simulink model "GFM_parallel_alt"  (R2024a)
settings: Solver=VariableStepAuto  StartTime=0.0  StopTime=40  FixedStep=5e-6  RelTol=1e-3
values from neighbouring files (symbols this model uses):
  Cf_pu = 0.03    [main__gfm.m]    (also in main_parallel.m; main_parallel_alt.m; main_standalone.m; scr.m)
  Cs_pu = 0.3    [main_parallel.m]    (also in main_parallel_alt.m; main_standalone.m)
  Dp = 0.02    [main__gfm.m]    (also in main_parallel.m; main_parallel_alt.m; main_standalone.m; scr.m)
  Dp1 = Dp    (= 0.02)    [main_parallel.m]    (also in main_parallel_alt.m)
  Dp2 = Dp    (= 0.02)    [main_parallel.m]    (also in main_parallel_alt.m)
  Dq = 0.3    [main__gfm.m]    (also in main_parallel.m; main_parallel_alt.m; main_standalone.m; scr.m)
  Dq1 = Dq    (= 0.3)    [main_parallel.m]    (also in main_parallel_alt.m)
  Dq2 = Dq    (= 0.3)    [main_parallel.m]    (also in main_parallel_alt.m)
  fac = 0    [main__gfm.m]    (also in main_parallel.m; main_parallel_alt.m; main_standalone.m; scr.m)
  H = 1.2    [main__gfm.m]    (also in main_parallel.m = 0.3; main_parallel_alt.m = 0.3; main_standalone.m; scr.m)
  I_load = Vpcc0/Zload_pu    [main__gfm.m]    (also in main_parallel.m = Vpcc/Zload_pu; main_parallel_alt.m = Vpoc/Zload_pu; main_standalone.m; scr.m)
  Ic1 = (Vconv1-Vlcl1)/(Rc_pu+1i*Lc_pu)    [main_parallel.m]    (also in main_parallel_alt.m = (Vconv1-Vpcc1)/(Rc_pu+1i*Lc_pu))
  Ic2 = (Vconv2-Vlcl2)/(Rc_pu+1i*Lc_pu)    [main_parallel.m]    (also in main_parallel_alt.m = (Vconv2-Vpcc2)/(Rc_pu+1i*Lc_pu))
  If1 = (Vlcl1-Vpcc)/(Rgf_pu+1i*Lgf_pu)    [main_parallel.m]    (also in main_parallel_alt.m = (Vpcc1-Vpoc)/(Rgf_pu+1i*Lgf_pu))
  If2 = (Vlcl2-Vpcc)/(Rgf_pu+1i*Lgf_pu)    [main_parallel.m]    (also in main_parallel_alt.m = (Vpcc2-Vpoc)/(Rgf_pu+1i*Lgf_pu))
  Iinf = (Vpcc-Vinf)/(Rgrid_pu+1i*Lgrid_pu)    [main_parallel.m]    (also in main_parallel_alt.m = (Vpoc-Vinf)/(Rgrid_pu+1i*Lgrid_pu))
  Kd = 50    [main__gfm.m]    (also in main_parallel.m; main_parallel_alt.m = 100; main_standalone.m; scr.m)
  kfi = 0    [main__gfm.m]    (also in main_parallel.m; main_parallel_alt.m; main_standalone.m; scr.m)
  kii = Rc_pu / L * kpi    [main__gfm.m]    (also in main_parallel.m; main_parallel_alt.m; main_standalone.m; scr.m)
  kiq = 0.1    [main__gfm.m]    (also in main_parallel.m = 0.01; main_parallel_alt.m = 0.01; main_standalone.m; scr.m)
  kivd = 100    [main__gfm.m]    (also in main_parallel.m = 50; main_parallel_alt.m = 50; main_standalone.m; scr.m)
  kivq = 100    [main__gfm.m]    (also in main_parallel.m = 50; main_parallel_alt.m = 50; main_standalone.m; scr.m)
  kpi = 2 * pi * f_bw * L    [main__gfm.m]    (also in main_parallel.m; main_parallel_alt.m; main_standalone.m; scr.m)
  kpvd = 0.1    [main__gfm.m]    (also in main_parallel.m = 0.45; main_parallel_alt.m = 0.45; main_standalone.m; scr.m)
  kpvq = 0.1    [main__gfm.m]    (also in main_parallel.m = 0.45; main_parallel_alt.m = 0.45; main_standalone.m; scr.m = 1)
  Lc_pu = Lc / Lb    [main__gfm.m]    (also in main_parallel.m; main_parallel_alt.m; main_standalone.m; scr.m)
  Lgf_pu = Lgf/Lb    (= 0.0166666666667)    [main_parallel.m]    (also in main_parallel_alt.m; main_standalone.m)
  Lgrid_pu = 1    [main_parallel.m]    (also in main_parallel_alt.m)
  Pref1 = -line_flow(7,4)    [main_parallel.m]    (also in main_parallel_alt.m)
  Pref2 = -line_flow(3,4)    [main_parallel.m]    (also in main_parallel_alt.m)
  PsiId1 = real(Vconv_c1)-real(Vpcc_c)+X*imag(Ifc1)    [main_parallel.m]    (also in main_parallel_alt.m)
  PsiId2 = real(Vconv_c2)-real(Vpcc_c)+X*imag(Ifc2)    [main_parallel.m]    (also in main_parallel_alt.m)
  PsiIq1 = imag(Vconv_c1)-imag(Vpcc_c)-X*real(Ifc1)    [main_parallel.m]    (also in main_parallel_alt.m)
  PsiIq2 = imag(Vconv_c2)-imag(Vpcc_c)-X*real(Ifc2)    [main_parallel.m]    (also in main_parallel_alt.m)
  PsiP1 = real(Ifc1)-wCpu*imag(Vpcc_c)*fac+imag(Ifc1)*kfi    [main_parallel.m]    (also in main_parallel_alt.m)
  PsiP2 = real(Ifc2)-wCpu*imag(Vpcc_c)*fac+imag(Ifc2)*kfi    [main_parallel.m]    (also in main_parallel_alt.m)
  PsiV1 = imag(Ifc1)+wCpu*real(Vpcc_c)*fac+real(Ifc1)*kfi    [main_parallel.m]    (also in main_parallel_alt.m)
  PsiV2 = imag(Ifc2)+wCpu*real(Vpcc_c)*fac+real(Ifc2)*kfi    [main_parallel.m]    (also in main_parallel_alt.m)
  Qref1 = -line_flow(7,5)    [main_parallel.m]    (also in main_parallel_alt.m)
  Qref2 = -line_flow(3,5)    [main_parallel.m]    (also in main_parallel_alt.m)
  Rc_pu = Rc / Zb    (= 5.19390581717e-06)    [main__gfm.m]    (also in main_parallel.m; main_parallel_alt.m; main_standalone.m; scr.m)
  Rf_pu = Rf / Zb    [main__gfm.m]    (also in main_parallel.m; main_parallel_alt.m; main_standalone.m; scr.m)
  Rgf_pu = 0    [main_parallel.m]    (also in main_parallel_alt.m)
  Rgrid_pu = Lgrid_pu*XrXg    (= 0)    [main_parallel.m]    (also in main_parallel_alt.m)
  Rs_pu = 0.1    [main_parallel.m]    (also in main_parallel_alt.m; main_standalone.m)
  theta_ref = theta(2,1)    [main__gfm.m]    (also in main_parallel.m = theta(3,1); main_parallel_alt.m = theta(3,1); main_standalone.m = theta(3,1); scr.m)
  Vcf1 = Vlcl1+ Rf_pu*Icf1    [main_parallel.m]    (also in main_parallel_alt.m = Vpcc1+ Rf_pu*Icf1)
  Vcf2 = Vlcl2+ Rf_pu*Icf2    [main_parallel.m]    (also in main_parallel_alt.m = Vpcc2+ Rf_pu*Icf2)
  Vconv1 = V0(1,1)    [main_parallel.m]    (also in main_parallel_alt.m)
  Vconv_c1 = Vconv1 * exp(-1i*theta_ref)    [main_parallel.m]    (also in main_parallel_alt.m)
  Vconv_c2 = Vconv2 * exp(-1i*theta_ref)    [main_parallel.m]    (also in main_parallel_alt.m)
  Vinf = V0(3,1)    [main__gfm.m]    (also in main_parallel.m = V0(6,1); main_parallel_alt.m = V0(6,1); main_standalone.m = V0(4,1); scr.m)
  Vpcc = V0(3,1)    [main_parallel.m]
  Vs = Vpcc + Rs_pu*Igf    [main_parallel.m]    (also in main_parallel_alt.m = Vpoc + Rs_pu*Igf; main_standalone.m = Vload+Rs_pu*Ibf)
  wCpu = Zb * wb * Cf    (= 0.03)    [main__gfm.m]    (also in main_parallel.m; main_parallel_alt.m; main_standalone.m; scr.m)
  wLpu = X    [main__gfm.m]    (also in main_parallel.m; main_parallel_alt.m; main_standalone.m; scr.m)
  Zload_pu = inv(YL(2,2))    [main__gfm.m]    (also in main_parallel.m = inv(YL(3,3)); main_parallel_alt.m = inv(YL(3,3)); main_standalone.m = inv(YL(3,3)); scr.m)
undefined symbols (not defined in the file or in its folder): md, nd
settings Model: Creator=HP  LastModifiedBy=HP

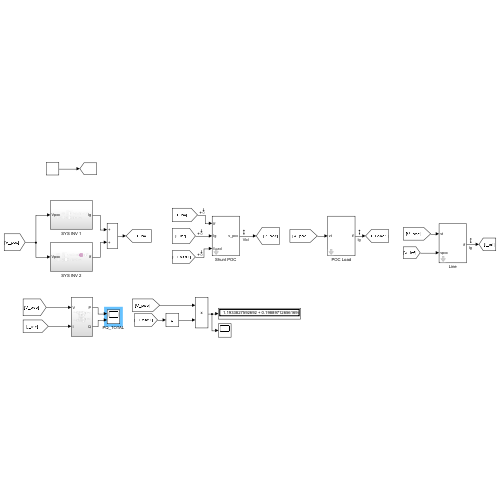
[thumbnail: Simulink's stored preview of the top-level diagram]
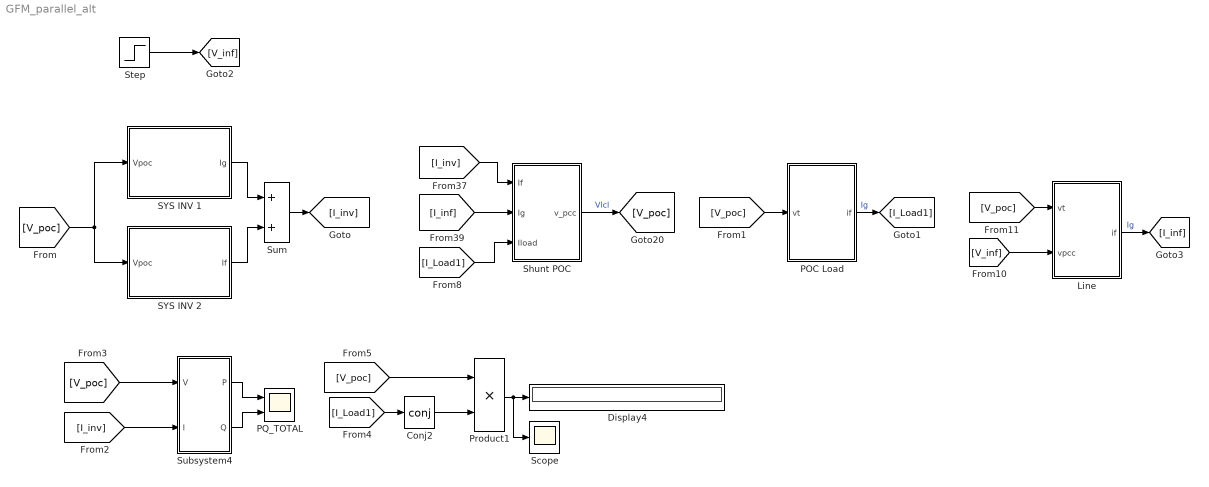
== system GFM_parallel_alt ==
  Conj2 : Math  Operator=conj
  Display4 : Display
  Line : Subsystem  mask{i0=Iinf, R=Rgrid_pu, L=Lgrid_pu}
      mask prompts: i0 "I initial condition (pu)"; R "R (pu)"; L "L (pu)"
  POC Load : Subsystem  mask{i0=I_load, R=real(Zload_pu), L=imag(Zload_pu)}
      mask prompts: i0 "I initial condition (pu)"; R "R (pu)"; L "L (pu)"
  PQ_TOTAL : Scope  NumInputPorts=2
  Product1 : Product
  SYS INV 1 : Subsystem
  SYS INV 2 : Subsystem
  Scope : Scope
  Shunt POC : Subsystem  mask{vc0=Vs, R=Rs_pu, C=Cs_pu}
      mask prompts: vc0 "initial value Vpcc  (p.u.)"; R "R (pu)"; C "C (pu)"
  Step : Step  Before=Vinf  After=Vinf  SampleTime=0
  Subsystem4 : Subsystem
  Sum : Sum
  wires:
  Step/1 -> [V_inf]
  [V_poc] -> Subsystem4/1(V)
  Subsystem4/2(Q) -> PQ_TOTAL/2
  [I_Load1] -> Conj2/1
  Product1/1 -> Scope/1, Display4/1
  Subsystem4/1(P) -> PQ_TOTAL/1
  [V_poc] -> Product1/1
  [I_inv] -> Subsystem4/2(I)
  [V_poc] -> SYS INV 1/1(Vpoc), SYS INV 2/1(Vpoc)
  [I_Load1] -> Shunt POC/3(Iload)
  [V_poc] -> Line/1("vt ")
  SYS INV 1/1(Ig) -> Sum/1
  POC Load/1(if) -> [I_Load1]  "Ig"
  [I_inf] -> Shunt POC/2("Ig ")
  [V_inf] -> Line/2("vpcc ")
  Shunt POC/1(v_pcc) -> [V_poc]  "Vlcl"
  Conj2/1 -> Product1/2
  Sum/1 -> [I_inv]
  [V_poc] -> POC Load/1("vt ")
  [I_inv] -> Shunt POC/1("If ")
  Line/1(if) -> [I_inf]  "Ig"
  SYS INV 2/1(If) -> Sum/2

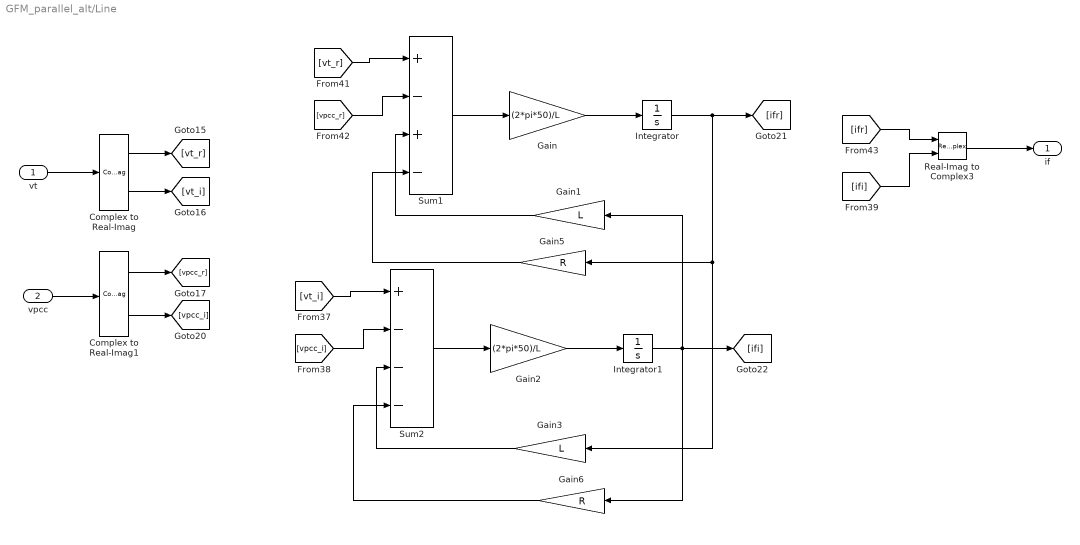
== system GFM_parallel_alt/Line ==
  "vt " : Inport
  "vpcc " : Inport  Port=2
  Complex to Real-Imag : ComplexToRealImag
  Complex to Real-Imag1 : ComplexToRealImag
  Gain : Gain  Gain=(2*pi*50)/L
  Gain1 : Gain  Gain=L
  Gain2 : Gain  Gain=(2*pi*50)/L
  Gain3 : Gain  Gain=L
  Gain5 : Gain  Gain=R
  Gain6 : Gain  Gain=R
  Integrator : Integrator  InitialCondition=real(i0)  ContinuousStateAttributes='Iline_re'
  Integrator1 : Integrator  InitialCondition=imag(i0)  ContinuousStateAttributes='iline_im'
  Real-Imag to Complex3 : RealImagToComplex
  Sum1 : Sum  Inputs=+-+-
  Sum2 : Sum  Inputs=+---
  if : Outport
  wires:
  "vpcc "/1 -> Complex to Real-Imag1/1
  Gain5/1 -> Sum1/4
  Real-Imag to Complex3/1 -> if/1
  Integrator1/1 -> Gain6/1, Gain1/1, [ifi]
  [ifr] -> Real-Imag to Complex3/1
  "vt "/1 -> Complex to Real-Imag/1
  Integrator/1 -> Gain5/1, Gain3/1, [ifr]
  [ifi] -> Real-Imag to Complex3/2
  [vpcc_r] -> Sum1/2
  Gain6/1 -> Sum2/4
  Complex to Real-Imag/1 -> [vt_r]
  Gain1/1 -> Sum1/3
  Complex to Real-Imag/2 -> [vt_i]
  Complex to Real-Imag1/1 -> [vpcc_r]
  Sum2/1 -> Gain2/1
  Gain2/1 -> Integrator1/1
  [vt_i] -> Sum2/1
  [vpcc_i] -> Sum2/2
  [vt_r] -> Sum1/1
  Gain3/1 -> Sum2/3
  Complex to Real-Imag1/2 -> [vpcc_i]
  Gain/1 -> Integrator/1
  Sum1/1 -> Gain/1

== system GFM_parallel_alt/POC Load ==
  "vt " : Inport
  Complex to Real-Imag : ComplexToRealImag
  Gain : Gain  Gain=(2*pi*50)/L
  Gain1 : Gain  Gain=L
  Gain2 : Gain  Gain=(2*pi*50)/L
  Gain3 : Gain  Gain=L
  Gain5 : Gain  Gain=R
  Gain6 : Gain  Gain=R
  Integrator : Integrator  InitialCondition=real(i0)  ContinuousStateAttributes='iload_re'
  Integrator1 : Integrator  InitialCondition=imag(i0)  ContinuousStateAttributes='load_im'
  Real-Imag to Complex3 : RealImagToComplex
  Sum1 : Sum  Inputs=+-+-
  Sum2 : Sum  Inputs=+---
  if : Outport
  wires:
  Gain5/1 -> Sum1/4
  Real-Imag to Complex3/1 -> if/1
  Integrator1/1 -> Gain6/1, Gain1/1, [ifi]
  [ifr] -> Real-Imag to Complex3/1
  "vt "/1 -> Complex to Real-Imag/1
  Integrator/1 -> Gain5/1, Gain3/1, [ifr]
  [ifi] -> Real-Imag to Complex3/2
  Gain6/1 -> Sum2/4
  Complex to Real-Imag/1 -> [vt_r]
  Gain1/1 -> Sum1/3
  Complex to Real-Imag/2 -> [vt_i]
  Sum2/1 -> Gain2/1
  Gain2/1 -> Integrator1/1
  [vt_i] -> Sum2/1
  [vt_r] -> Sum1/1
  Gain3/1 -> Sum2/3
  Gain/1 -> Integrator/1
  Sum1/1 -> Gain/1

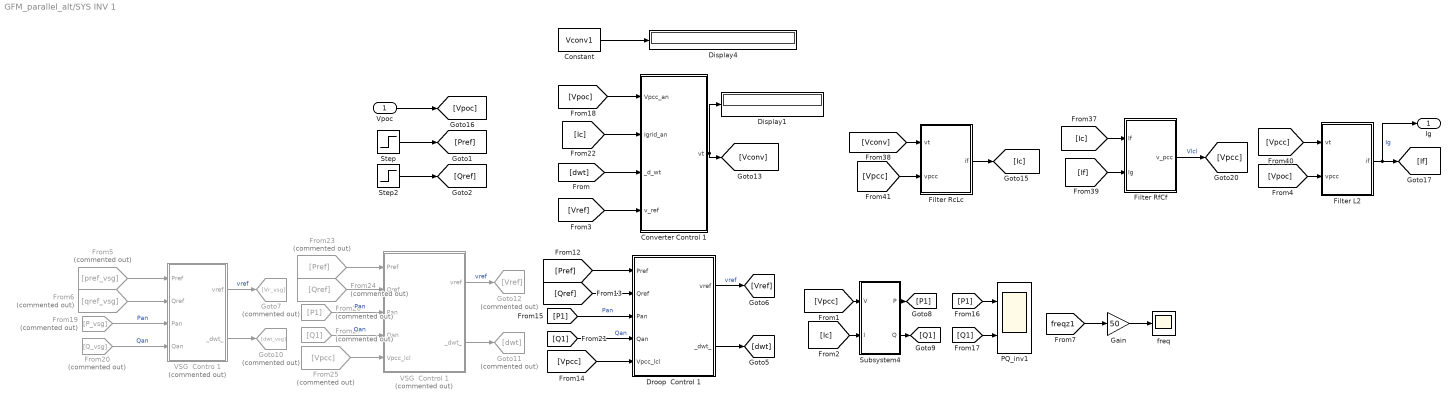
== system GFM_parallel_alt/SYS INV 1 ==
  Vpoc : Inport
  Constant : Constant  Value=Vconv1
  Converter Control 1 : Subsystem
  Display1 : Display
  Display4 : Display
  Droop  Control 1 : Subsystem  mask{kiq=0, md=Dp1, nd=Dq1, wt0=theta_ref, vref_=Vpcc}
      mask prompts: kiq "KiQ-V"; md "P droop"; nd "Qdroop"; wt0 "initial theta"; vref_ "Voltage ref"
  Filter L2 : Subsystem  mask{i0=If1, R=Rgf_pu, L=Lgf_pu}
      mask prompts: i0 "I initial condition (pu)"; R "R (pu)"; L "L (pu)"
  Filter RcLc : Subsystem  mask{i0=Ic1, R=Rc_pu, L=Lc_pu}
      mask prompts: i0 "I initial condition (pu)"; R "R (pu)"; L "L (pu)"
  Filter RfCf : Subsystem  mask{vc0=Vcf1, R=Rf_pu, C=Cf_pu}
      mask prompts: vc0 "initial value Vpcc  (p.u.)"; R "R (pu)"; C "C (pu)"
  From19 : From  Commented=on  GotoTag=P_vsg
  From20 : From  Commented=on  GotoTag=Q_vsg
  From23 : From  Commented=on  GotoTag=Pref
  From24 : From  Commented=on  GotoTag=Qref
  From25 : From  Commented=on  GotoTag=Vpcc
  From26 : From  Commented=on  GotoTag=P1
  From27 : From  Commented=on  GotoTag=Q1
  From5 : From  Commented=on  GotoTag=pref_vsg
  From6 : From  Commented=on  GotoTag=qref_vsg
  Gain : Gain  Gain=50
  Goto10 : Goto  Commented=on  GotoTag=dwt_vsg
  Goto11 : Goto  Commented=on  GotoTag=dwt
  Goto12 : Goto  Commented=on  GotoTag=Vref
  Goto7 : Goto  Commented=on  GotoTag=Vr_vsg
  PQ_inv1 : Scope  NumInputPorts=2
  Step : Step  Before=Pref1  After=0.5  SampleTime=0
  Step2 : Step  Before=Qref1  After=0.1  SampleTime=0
  Subsystem4 : Subsystem
  VSG  Contro 1 : Subsystem  Commented=on  mask{kip=0, kiq=6, md=md, nd=nd, wt0=theta_ref, vref_=Vpcc, H=0.4}
      mask prompts: kip "KiP-W"; kiq "KiQ-V"; md "P droop"; nd "Qdroop"; wt0 "initial theta"; vref_ "Voltage ref"; H "H (inertia constant)"
  VSG  Control 1 : Subsystem  Commented=on  mask{kiq=kiq, Kd=Kd, nd=Dq1, H=H, wt0=theta_ref, vref_=Vpcc}
      mask prompts: kiq "KiQ-V"; Kd "Damping Factor"; nd "Q droop"; H "Inertia Constant"; wt0 "initial theta"; vref_ "Voltage ref"
  freq : Scope
  Ig : Outport
  wires:
  [Ic] -> Converter Control 1/2(Igrid_an)
  [Ic] -> Subsystem4/2(I)
  From19/1 -> VSG  Contro 1/3(Pan)  "Pan"
  Filter L2/1(if) -> Ig/1, [If]  "Ig"
  [If] -> Filter RfCf/2("Ig ")
  Filter RfCf/1(v_pcc) -> [Vpcc]  "Vlcl"
  Converter Control 1/1(vt) -> [Vconv], Display1/1
  [dwt] -> Converter Control 1/3(_d_wt)
  Gain/1 -> freq/1
  Subsystem4/2(Q) -> [Q1]
  [P1] -> PQ_inv1/1
  From20/1 -> VSG  Contro 1/4(Qan)  "Qan"
  [Ic] -> Filter RfCf/1("If ")
  [Vpcc] -> Filter RcLc/2("vpcc ")
  [Vconv] -> Filter RcLc/1("vt ")
  [Vref] -> Converter Control 1/4(v_ref)
  [freqz1] -> Gain/1
  [Q1] -> PQ_inv1/2
  From5/1 -> VSG  Contro 1/1(Pref)
  Filter RcLc/1(if) -> [Ic]
  [Vpcc] -> Subsystem4/1(V)
  Subsystem4/1(P) -> [P1]
  [Vpcc] -> Filter L2/1("vt ")
  [Vpoc] -> Converter Control 1/1(Vpcc_an)
  VSG  Contro 1/2(_dwt_) -> Goto10/1
  Step2/1 -> [Qref]
  Step/1 -> [Pref]
  VSG  Contro 1/1(vref) -> Goto7/1  "vref"
  From6/1 -> VSG  Contro 1/2(Qref)
  [Vpoc] -> Filter L2/2("vpcc ")
  Vpoc/1 -> [Vpoc]
  Constant/1 -> Display4/1
  VSG  Control 1/1(vref) -> Goto12/1  "vref"
  From25/1 -> VSG  Control 1/5(Vpcc_lcl)
  VSG  Control 1/2(_dwt_) -> Goto11/1
  From23/1 -> VSG  Control 1/1(Pref)
  From24/1 -> VSG  Control 1/2(Qref)
  From26/1 -> VSG  Control 1/3(Pan)  "Pan"
  From27/1 -> VSG  Control 1/4(Qan)  "Qan"
  [Q1] -> Droop  Control 1/4(Qan)  "Qan"
  Droop  Control 1/2(_dwt_) -> [dwt]
  [Qref] -> Droop  Control 1/2(Qref)
  [P1] -> Droop  Control 1/3(Pan)  "Pan"
  [Pref] -> Droop  Control 1/1(Pref)
  Droop  Control 1/1(vref) -> [Vref]  "vref"
  [Vpcc] -> Droop  Control 1/5(Vpcc_lcl)

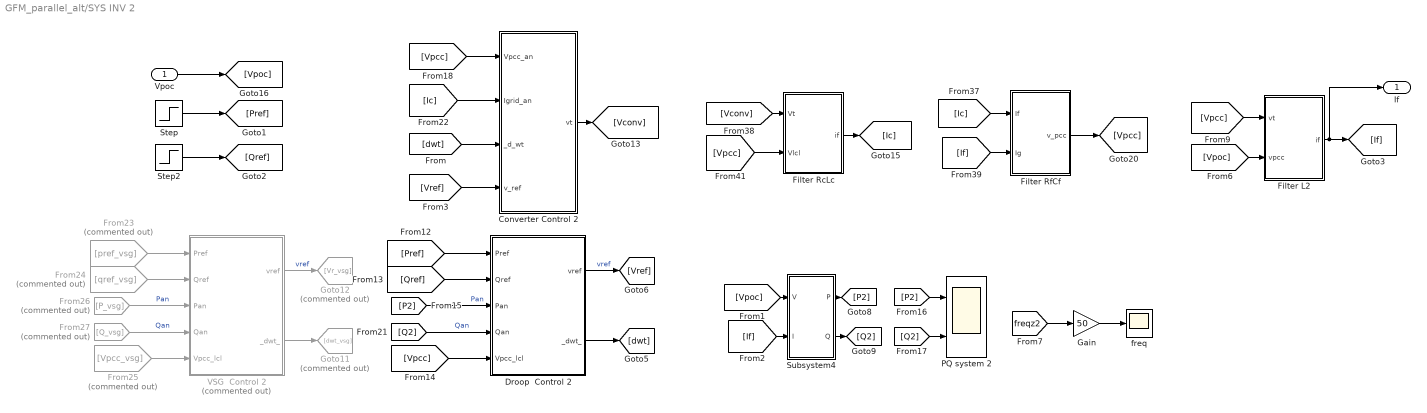
== system GFM_parallel_alt/SYS INV 2 ==
  Vpoc : Inport
  Converter Control 2 : Subsystem
  Droop  Control 2 : Subsystem  mask{kiq=0, md=Dp2, nd=Dq2, wt0=theta_ref, vref_=Vpcc}
      mask prompts: kiq "KiQ-V"; md "P droop"; nd "Qdroop"; wt0 "initial theta"; vref_ "Voltage ref"
  Filter L2 : Subsystem  mask{i0=If2, R=Rgf_pu, L=Lgf_pu}
      mask prompts: i0 "I initial condition (pu)"; R "R (pu)"; L "L (pu)"
  Filter RcLc : Subsystem  mask{i0=Ic2, R=Rc_pu, L=Lc_pu}
      mask prompts: i0 "I initial condition (pu)"; R "R (pu)"; L "L (pu)"
  Filter RfCf : Subsystem  mask{vc0=Vcf2, R=Rf_pu, C=Cf_pu}
      mask prompts: vc0 "initial value Vpcc  (p.u.)"; R "R (pu)"; C "C (pu)"
  From23 : From  Commented=on  GotoTag=pref_vsg
  From24 : From  Commented=on  GotoTag=qref_vsg
  From25 : From  Commented=on  GotoTag=Vpcc_vsg
  From26 : From  Commented=on  GotoTag=P_vsg
  From27 : From  Commented=on  GotoTag=Q_vsg
  Gain : Gain  Gain=50
  Goto11 : Goto  Commented=on  GotoTag=dwt_vsg
  Goto12 : Goto  Commented=on  GotoTag=Vr_vsg
  PQ system 2 : Scope  NumInputPorts=2
  Step : Step  Before=Pref2  After=0.3  SampleTime=0
  Step2 : Step  Before=Qref2  After=0.1  SampleTime=0
  Subsystem4 : Subsystem
  VSG  Control 2 : Subsystem  Commented=on  mask{kiq=kiq, md=Dp, nd=Dq, H=H, wt0=theta_ref, vref_=Vpcc}
      mask prompts: kiq "KiQ-V"; md "P droop, damp fact (1/md)"; nd "Q droop"; H "Inertia Constant"; wt0 "initial theta"; vref_ "Voltage ref"
  freq : Scope
  If : Outport
  wires:
  [Ic] -> Converter Control 2/2(Igrid_an)
  [If] -> Subsystem4/2(I)
  [If] -> Filter RfCf/2("Ig ")
  Filter RfCf/1(v_pcc) -> [Vpcc]
  Converter Control 2/1(vt) -> [Vconv]
  [dwt] -> Converter Control 2/3(_d_wt)
  Gain/1 -> freq/1
  Subsystem4/2(Q) -> [Q2]
  [P2] -> PQ system 2/1
  [Ic] -> Filter RfCf/1("If ")
  [Vpcc] -> Filter RcLc/2("Vlcl ")
  [Vconv] -> Filter RcLc/1("Vt ")
  [Vref] -> Converter Control 2/4(v_ref)
  [freqz2] -> Gain/1
  [Q2] -> PQ system 2/2
  Filter RcLc/1(if) -> [Ic]
  [Vpoc] -> Subsystem4/1(V)
  Subsystem4/1(P) -> [P2]
  [Vpcc] -> Converter Control 2/1(Vpcc_an)
  Step2/1 -> [Qref]
  Step/1 -> [Pref]
  Vpoc/1 -> [Vpoc]
  [P2] -> Droop  Control 2/3(Pan)  "Pan"
  [Qref] -> Droop  Control 2/2(Qref)
  [Vpcc] -> Droop  Control 2/5(Vpcc_lcl)
  Droop  Control 2/2(_dwt_) -> [dwt]
  [Q2] -> Droop  Control 2/4(Qan)  "Qan"
  [Pref] -> Droop  Control 2/1(Pref)
  Droop  Control 2/1(vref) -> [Vref]  "vref"
  From27/1 -> VSG  Control 2/4(Qan)  "Qan"
  From26/1 -> VSG  Control 2/3(Pan)  "Pan"
  From23/1 -> VSG  Control 2/1(Pref)
  From24/1 -> VSG  Control 2/2(Qref)
  From25/1 -> VSG  Control 2/5(Vpcc_lcl)
  VSG  Control 2/1(vref) -> Goto12/1  "vref"
  VSG  Control 2/2(_dwt_) -> Goto11/1
  [Vpcc] -> Filter L2/1("vt ")
  Filter L2/1(if) -> If/1, [If]
  [Vpoc] -> Filter L2/2("vpcc ")

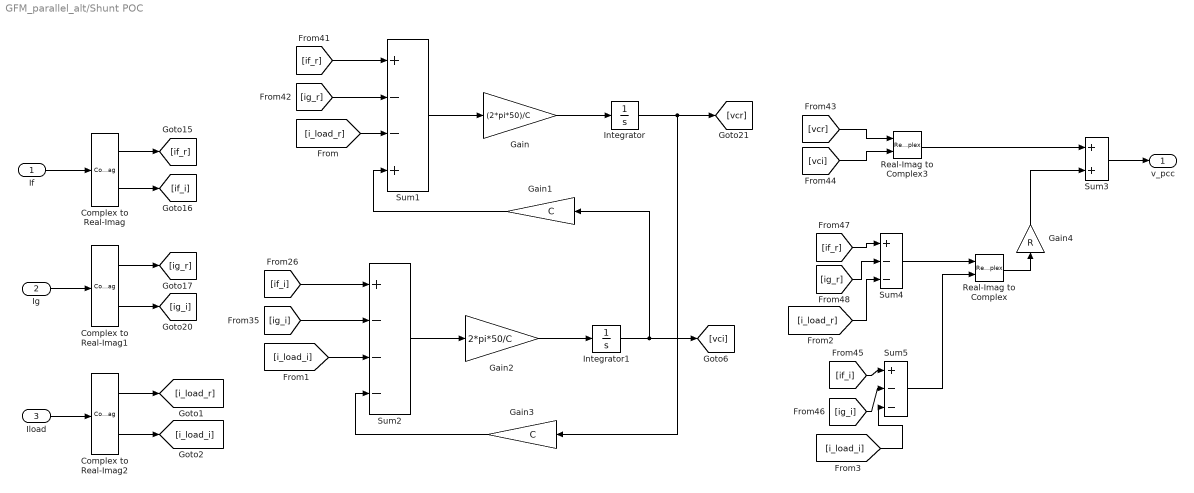
== system GFM_parallel_alt/Shunt POC ==
  "If " : Inport
  "Ig " : Inport  Port=2
  Iload : Inport  Port=3
  Complex to Real-Imag : ComplexToRealImag
  Complex to Real-Imag1 : ComplexToRealImag
  Complex to Real-Imag2 : ComplexToRealImag
  Gain : Gain  Gain=(2*pi*50)/C
  Gain1 : Gain  Gain=C
  Gain2 : Gain  Gain=2*pi*50/C
  Gain3 : Gain  Gain=C
  Gain4 : Gain  Gain=R
  Integrator : Integrator  InitialCondition=real(vc0)  ContinuousStateAttributes='vc_par_re'
  Integrator1 : Integrator  InitialCondition=imag(vc0)  ContinuousStateAttributes='vc_par_im'
  Real-Imag to Complex : RealImagToComplex
  Real-Imag to Complex3 : RealImagToComplex
  Sum1 : Sum  Inputs=+--+
  Sum2 : Sum  Inputs=+---
  Sum3 : Sum
  Sum4 : Sum  Inputs=+--
  Sum5 : Sum  Inputs=+--
  v_pcc : Outport
  wires:
  Sum4/1 -> Real-Imag to Complex/1
  "Ig "/1 -> Complex to Real-Imag1/1
  Complex to Real-Imag1/2 -> [ig_i]
  Integrator1/1 -> Gain1/1, [vci]
  Sum1/1 -> Gain/1
  Gain/1 -> Integrator/1
  [ig_r] -> Sum1/2
  Real-Imag to Complex/1 -> Gain4/1
  [ig_r] -> Sum4/2
  [ig_i] -> Sum5/2
  Integrator/1 -> Gain3/1, [vcr]
  [ig_i] -> Sum2/2
  Gain2/1 -> Integrator1/1
  "If "/1 -> Complex to Real-Imag/1
  [if_i] -> Sum2/1
  [if_r] -> Sum4/1
  Sum2/1 -> Gain2/1
  [if_r] -> Sum1/1
  Sum5/1 -> Real-Imag to Complex/2
  Sum3/1 -> v_pcc/1
  [if_i] -> Sum5/1
  Gain4/1 -> Sum3/2
  Complex to Real-Imag/2 -> [if_i]
  [vci] -> Real-Imag to Complex3/2
  Real-Imag to Complex3/1 -> Sum3/1
  Complex to Real-Imag1/1 -> [ig_r]
  Complex to Real-Imag/1 -> [if_r]
  [vcr] -> Real-Imag to Complex3/1
  Gain1/1 -> Sum1/4
  Gain3/1 -> Sum2/4
  Complex to Real-Imag2/1 -> [i_load_r]
  Complex to Real-Imag2/2 -> [i_load_i]
  Iload/1 -> Complex to Real-Imag2/1
  [i_load_r] -> Sum1/3
  [i_load_i] -> Sum2/3
  [i_load_r] -> Sum4/3
  [i_load_i] -> Sum5/3

== system GFM_parallel_alt/Subsystem4 ==
  V : Inport
  I : Inport  Port=2
  Complex to Real-Imag : ComplexToRealImag
  Complex to Real-Imag1 : ComplexToRealImag
  Product{,1..3} (4 alike) : Product
  Sum : Sum
  Sum1 : Sum  Inputs=-+
  P : Outport
  Q : Outport  Port=2
  wires:
  Complex to Real-Imag/1 -> Product2/1, Product/1
  Sum1/1 -> Q/1
  V/1 -> Complex to Real-Imag/1
  Complex to Real-Imag1/2 -> Product2/2, Product1/2
  Product1/1 -> Sum/2
  Sum/1 -> P/1
  I/1 -> Complex to Real-Imag1/1
  Complex to Real-Imag/2 -> Product3/1, Product1/1
  Complex to Real-Imag1/1 -> Product/2, Product3/2
  Product/1 -> Sum/1
  Product3/1 -> Sum1/2
  Product2/1 -> Sum1/1

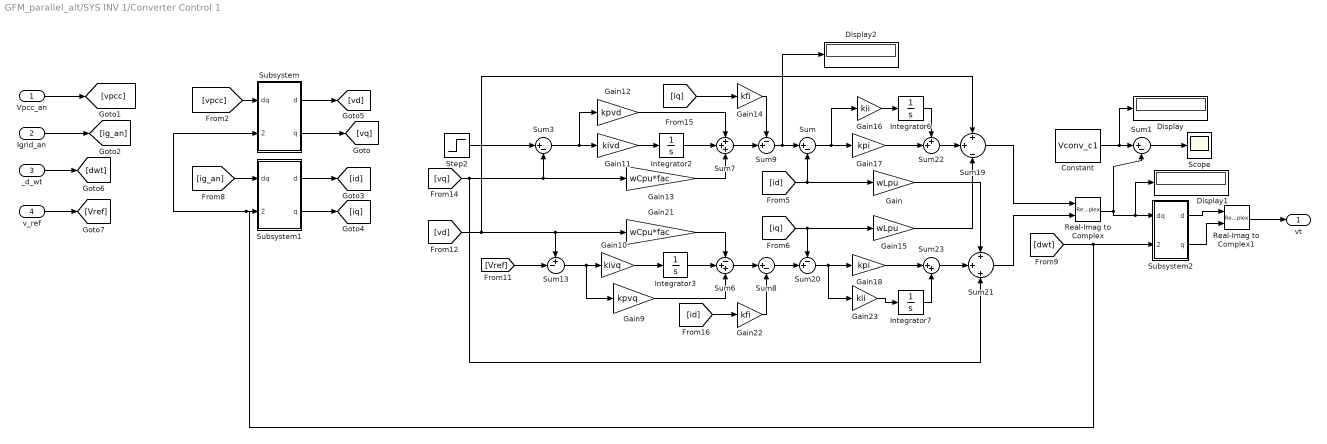
== system GFM_parallel_alt/SYS INV 1/Converter Control 1 ==
  Vpcc_an : Inport
  Igrid_an : Inport  Port=2
  _d_wt : Inport  Port=3
  v_ref : Inport  Port=4
  Constant : Constant  Value=Vconv_c1
  Display : Display
  Display1 : Display
  Display2 : Display
  Gain : Gain  Gain=wLpu
  Gain10 : Gain  Gain=kivq
  Gain11 : Gain  Gain=kivd
  Gain12 : Gain  Gain=kpvd
  Gain13 : Gain  Gain=wCpu*fac
  Gain14 : Gain  Gain=kfi
  Gain15 : Gain  Gain=wLpu
  Gain16 : Gain  Gain=kii
  Gain17 : Gain  Gain=kpi
  Gain18 : Gain  Gain=kpi
  Gain21 : Gain  Gain=wCpu*fac
  Gain22 : Gain  Gain=kfi
  Gain23 : Gain  Gain=kii
  Gain9 : Gain  Gain=kpvq
  Integrator2 : Integrator  InitialCondition=PsiP1  ContinuousStateAttributes='psi_alpha1'
  Integrator3 : Integrator  InitialCondition=PsiV1  ContinuousStateAttributes='psiV1'
  Integrator6 : Integrator  InitialCondition=PsiId1  ContinuousStateAttributes='psi_id1'
  Integrator7 : Integrator  InitialCondition=PsiIq1  ContinuousStateAttributes='psi_iq1'
  Real-Imag to Complex : RealImagToComplex
  Real-Imag to Complex1 : RealImagToComplex
  Scope : Scope
  Step2 : Step  After=0  SampleTime=0
  Subsystem : Subsystem
  Subsystem1 : Subsystem
  Subsystem2 : Subsystem
  Sum{,1,3,8} (4 alike) : Sum  Inputs=|+-
  Sum13 : Sum  Inputs=+-|
  Sum19 : Sum  Inputs=+|+|-
  Sum20 : Sum  Inputs=-+|
  Sum21 : Sum  Inputs=+|+|+
  Sum22 : Sum  Inputs=++|
  Sum23 : Sum  Inputs=|++
  Sum6 : Sum  Inputs=-++
  Sum7 : Sum  Inputs=+++
  Sum9 : Sum  Inputs=-+|
  vt : Outport
  wires:
  Integrator3/1 -> Sum6/2
  Gain11/1 -> Integrator2/1
  Subsystem/2(q) -> [vq]
  Sum13/1 -> Gain10/1, Gain9/1
  Igrid_an/1 -> [ig_an]
  [vpcc] -> Subsystem/1(dq)
  Subsystem2/2(q) -> Real-Imag to Complex1/2
  Subsystem2/1(d) -> Real-Imag to Complex1/1
  [id] -> Sum/2, Gain/1
  Subsystem1/1(d) -> [id]
  [iq] -> Gain15/1, Sum20/1
  Sum21/1 -> Real-Imag to Complex/2
  Integrator6/1 -> Sum22/1
  Sum20/1 -> Gain23/1, Gain18/1
  Gain23/1 -> Integrator7/1
  Gain18/1 -> Sum23/1
  Sum22/1 -> Sum19/2
  Gain22/1 -> Sum8/2
  Gain10/1 -> Integrator3/1
  Gain14/1 -> Sum9/1
  Sum8/1 -> Sum20/2
  Sum7/1 -> Sum9/2
  [ig_an] -> Subsystem1/1(dq)
  Gain13/1 -> Sum7/3
  Sum19/1 -> Real-Imag to Complex/1
  Sum3/1 -> Gain12/1, Gain11/1
  Gain16/1 -> Integrator6/1
  Sum/1 -> Gain16/1, Gain17/1
  Gain/1 -> Sum21/1
  [Vref] -> Sum13/2
  Gain9/1 -> Sum6/3
  Gain21/1 -> Sum6/1
  Subsystem1/2(q) -> [iq]
  Integrator7/1 -> Sum23/2
  Sum23/1 -> Sum21/2
  Subsystem/1(d) -> [vd]
  [vq] -> Sum3/2, Gain13/1, Sum21/3
  Gain15/1 -> Sum19/3
  [vd] -> Gain21/1, Sum13/1, Sum19/1
  Gain17/1 -> Sum22/2
  [id] -> Gain22/1
  [iq] -> Gain14/1
  Vpcc_an/1 -> [vpcc]
  Gain12/1 -> Sum7/1
  Sum6/1 -> Sum8/1
  Integrator2/1 -> Sum7/2
  Real-Imag to Complex1/1 -> vt/1
  Sum9/1 -> Display2/1, Sum/1
  [dwt] -> Subsystem1/2(delta_wt), Subsystem/2(delta_wt), Subsystem2/2(d_wt)
  Step2/1 -> Sum3/1
  _d_wt/1 -> [dwt]
  v_ref/1 -> [Vref]
  Real-Imag to Complex/1 -> Display1/1, Subsystem2/1(dq), Sum1/2
  Constant/1 -> Display/1, Sum1/1
  Sum1/1 -> Scope/1

== system GFM_parallel_alt/SYS INV 1/Droop  Control 1 ==
  note: Q droop Outer Control
  note: P Droop Outer Control
  Pref : Inport
  Qref : Inport  Port=2
  Pan : Inport  Port=3
  Qan : Inport  Port=4
  Vpcc_lcl : Inport  Port=5
  Abs : Abs  SaturateOnIntegerOverflow=off
  Gain : Gain  Gain=kiq
  Gain13 : Gain  Gain=md
  Gain14 : Gain  Gain=nd
  Gain4 : Gain  Gain=2*pi*50
  Integrator : Integrator  InitialCondition=angle(vref_)  ContinuousStateAttributes='theta0_dr_1'
  Integrator1 : Integrator
  Step : Step  Before=1.00  After=1.000  SampleTime=0
  Step1 : Step  Before=abs(vref_)  After=abs(vref_)  SampleTime=0
  Step5 : Step  Time=2  Before=1  SampleTime=0
  Sum1 : Sum  Inputs=++|
  Sum12 : Sum  Inputs=++|
  Sum13 : Sum  Inputs=|+-
  Sum16 : Sum  Inputs=|+-
  Sum2 : Sum  Inputs=+-
  Sum3 : Sum  Inputs=++|
  vref : Outport
  _dwt_ : Outport  Port=2
  tag scope: freqz1=global
  wires:
  Gain13/1 -> Sum12/2
  Qref/1 -> Sum13/1
  Sum3/1 -> vref/1
  Qan/1 -> Sum13/2
  Pref/1 -> Sum16/1
  Pan/1 -> Sum16/2
  Sum13/1 -> Gain/1, Gain14/1
  Sum2/1 -> Gain4/1
  Gain4/1 -> Integrator/1
  Sum12/1 -> Sum2/1, [freqz1]
  Integrator/1 -> _dwt_/1
  Sum16/1 -> Gain13/1
  Step5/1 -> Sum12/1
  Step/1 -> Sum2/2
  Gain/1 -> Integrator1/1
  Gain14/1 -> Sum1/2
  Integrator1/1 -> Sum1/1
  Sum1/1 -> Sum3/2
  Vpcc_lcl/1 -> Abs/1
  Abs/1 -> [vpcc_abs]
  [vpcc_abs] -> Sum3/1

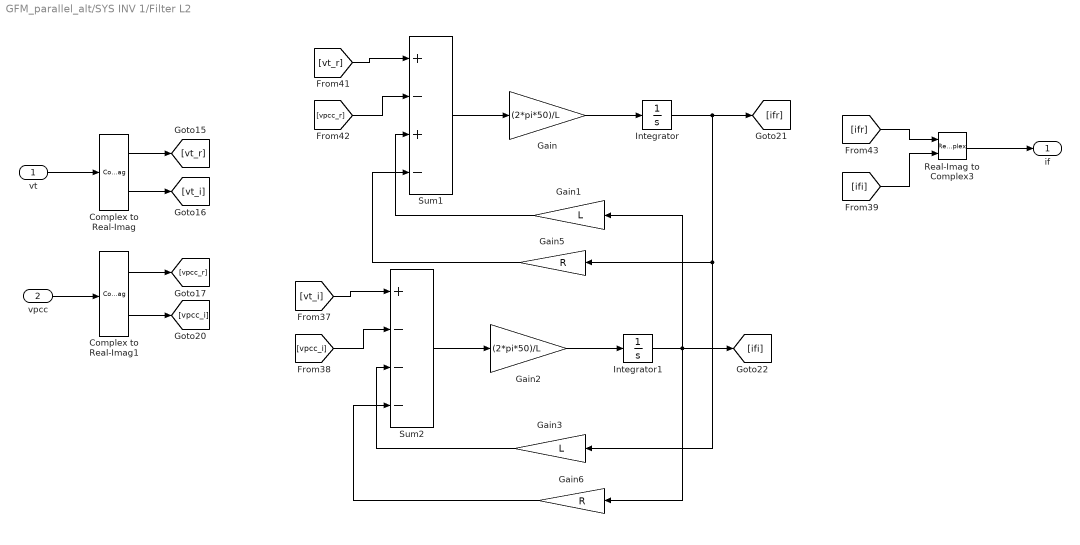
== system GFM_parallel_alt/SYS INV 1/Filter L2 ==
  "vt " : Inport
  "vpcc " : Inport  Port=2
  Complex to Real-Imag : ComplexToRealImag
  Complex to Real-Imag1 : ComplexToRealImag
  Gain : Gain  Gain=(2*pi*50)/L
  Gain1 : Gain  Gain=L
  Gain2 : Gain  Gain=(2*pi*50)/L
  Gain3 : Gain  Gain=L
  Gain5 : Gain  Gain=R
  Gain6 : Gain  Gain=R
  Integrator : Integrator  InitialCondition=real(i0)  ContinuousStateAttributes='ig1_re'
  Integrator1 : Integrator  InitialCondition=imag(i0)  ContinuousStateAttributes='ig1_im'
  Real-Imag to Complex3 : RealImagToComplex
  Sum1 : Sum  Inputs=+-+-
  Sum2 : Sum  Inputs=+---
  if : Outport
  wires:
  "vpcc "/1 -> Complex to Real-Imag1/1
  Gain5/1 -> Sum1/4
  Real-Imag to Complex3/1 -> if/1
  Integrator1/1 -> Gain6/1, Gain1/1, [ifi]
  [ifr] -> Real-Imag to Complex3/1
  "vt "/1 -> Complex to Real-Imag/1
  Integrator/1 -> Gain5/1, Gain3/1, [ifr]
  [ifi] -> Real-Imag to Complex3/2
  [vpcc_r] -> Sum1/2
  Gain6/1 -> Sum2/4
  Complex to Real-Imag/1 -> [vt_r]
  Gain1/1 -> Sum1/3
  Complex to Real-Imag/2 -> [vt_i]
  Complex to Real-Imag1/1 -> [vpcc_r]
  Sum2/1 -> Gain2/1
  Gain2/1 -> Integrator1/1
  [vt_i] -> Sum2/1
  [vpcc_i] -> Sum2/2
  [vt_r] -> Sum1/1
  Gain3/1 -> Sum2/3
  Complex to Real-Imag1/2 -> [vpcc_i]
  Gain/1 -> Integrator/1
  Sum1/1 -> Gain/1

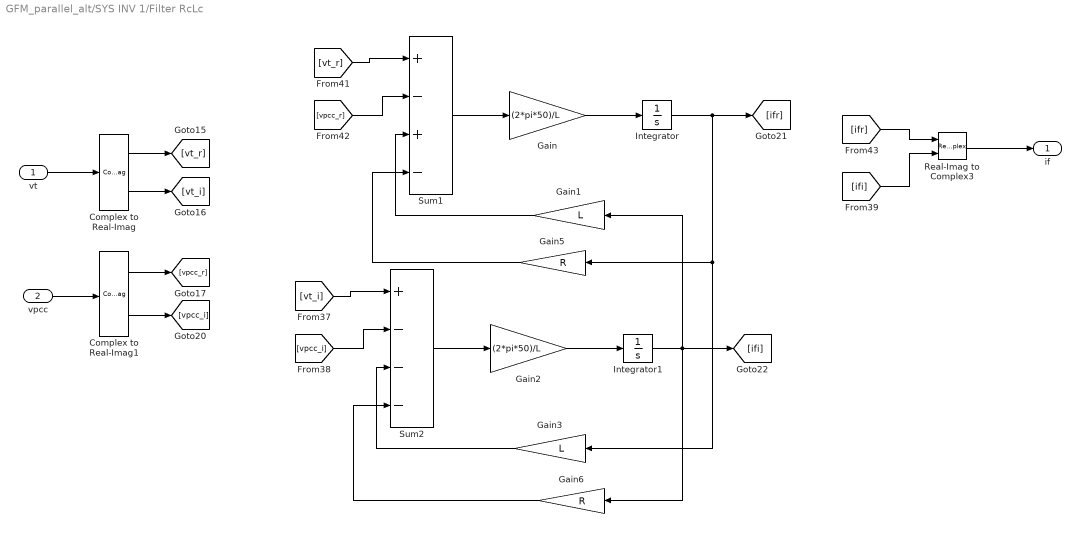
== system GFM_parallel_alt/SYS INV 1/Filter RcLc ==
  "vt " : Inport
  "vpcc " : Inport  Port=2
  Complex to Real-Imag : ComplexToRealImag
  Complex to Real-Imag1 : ComplexToRealImag
  Gain : Gain  Gain=(2*pi*50)/L
  Gain1 : Gain  Gain=L
  Gain2 : Gain  Gain=(2*pi*50)/L
  Gain3 : Gain  Gain=L
  Gain5 : Gain  Gain=R
  Gain6 : Gain  Gain=R
  Integrator : Integrator  InitialCondition=real(i0)  ContinuousStateAttributes='ic1_re'
  Integrator1 : Integrator  InitialCondition=imag(i0)  ContinuousStateAttributes='ic1_im'
  Real-Imag to Complex3 : RealImagToComplex
  Sum1 : Sum  Inputs=+-+-
  Sum2 : Sum  Inputs=+---
  if : Outport
  wires:
  "vpcc "/1 -> Complex to Real-Imag1/1
  Gain5/1 -> Sum1/4
  Real-Imag to Complex3/1 -> if/1
  Integrator1/1 -> Gain6/1, Gain1/1, [ifi]
  [ifr] -> Real-Imag to Complex3/1
  "vt "/1 -> Complex to Real-Imag/1
  Integrator/1 -> Gain5/1, Gain3/1, [ifr]
  [ifi] -> Real-Imag to Complex3/2
  [vpcc_r] -> Sum1/2
  Gain6/1 -> Sum2/4
  Complex to Real-Imag/1 -> [vt_r]
  Gain1/1 -> Sum1/3
  Complex to Real-Imag/2 -> [vt_i]
  Complex to Real-Imag1/1 -> [vpcc_r]
  Sum2/1 -> Gain2/1
  Gain2/1 -> Integrator1/1
  [vt_i] -> Sum2/1
  [vpcc_i] -> Sum2/2
  [vt_r] -> Sum1/1
  Gain3/1 -> Sum2/3
  Complex to Real-Imag1/2 -> [vpcc_i]
  Gain/1 -> Integrator/1
  Sum1/1 -> Gain/1

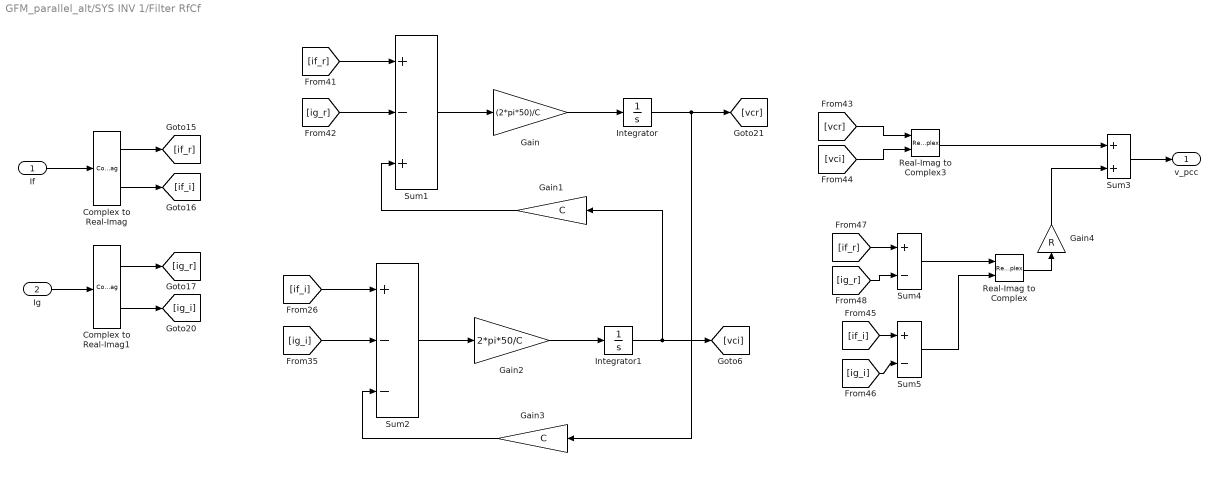
== system GFM_parallel_alt/SYS INV 1/Filter RfCf ==
  "If " : Inport
  "Ig " : Inport  Port=2
  Complex to Real-Imag : ComplexToRealImag
  Complex to Real-Imag1 : ComplexToRealImag
  Gain : Gain  Gain=(2*pi*50)/C
  Gain1 : Gain  Gain=C
  Gain2 : Gain  Gain=2*pi*50/C
  Gain3 : Gain  Gain=C
  Gain4 : Gain  Gain=R
  Integrator : Integrator  InitialCondition=real(vc0)  ContinuousStateAttributes='vc1_re'
  Integrator1 : Integrator  InitialCondition=imag(vc0)  ContinuousStateAttributes='vc1_im'
  Real-Imag to Complex : RealImagToComplex
  Real-Imag to Complex3 : RealImagToComplex
  Sum1 : Sum  Inputs=+-+
  Sum2 : Sum  Inputs=+--
  Sum3 : Sum
  Sum4 : Sum  Inputs=+-
  Sum5 : Sum  Inputs=+-
  v_pcc : Outport
  wires:
  Sum4/1 -> Real-Imag to Complex/1
  "Ig "/1 -> Complex to Real-Imag1/1
  Complex to Real-Imag1/2 -> [ig_i]
  Integrator1/1 -> Gain1/1, [vci]
  Sum1/1 -> Gain/1
  Gain/1 -> Integrator/1
  [ig_r] -> Sum1/2
  Real-Imag to Complex/1 -> Gain4/1
  Gain3/1 -> Sum2/3
  [ig_r] -> Sum4/2
  [ig_i] -> Sum5/2
  Integrator/1 -> Gain3/1, [vcr]
  [ig_i] -> Sum2/2
  Gain2/1 -> Integrator1/1
  "If "/1 -> Complex to Real-Imag/1
  [if_i] -> Sum2/1
  [if_r] -> Sum4/1
  Sum2/1 -> Gain2/1
  [if_r] -> Sum1/1
  Gain1/1 -> Sum1/3
  Sum5/1 -> Real-Imag to Complex/2
  Sum3/1 -> v_pcc/1
  [if_i] -> Sum5/1
  Gain4/1 -> Sum3/2
  Complex to Real-Imag/2 -> [if_i]
  [vci] -> Real-Imag to Complex3/2
  Real-Imag to Complex3/1 -> Sum3/1
  Complex to Real-Imag1/1 -> [ig_r]
  Complex to Real-Imag/1 -> [if_r]
  [vcr] -> Real-Imag to Complex3/1

== system GFM_parallel_alt/SYS INV 1/Subsystem4 ==
  V : Inport
  I : Inport  Port=2
  Complex to Real-Imag : ComplexToRealImag
  Complex to Real-Imag1 : ComplexToRealImag
  Product{,1..3} (4 alike) : Product
  Sum : Sum
  Sum1 : Sum  Inputs=-+
  P : Outport
  Q : Outport  Port=2
  wires:
  Complex to Real-Imag/1 -> Product2/1, Product/1
  Sum1/1 -> Q/1
  V/1 -> Complex to Real-Imag/1
  Complex to Real-Imag1/2 -> Product2/2, Product1/2
  Product1/1 -> Sum/2
  Sum/1 -> P/1
  I/1 -> Complex to Real-Imag1/1
  Complex to Real-Imag/2 -> Product3/1, Product1/1
  Complex to Real-Imag1/1 -> Product/2, Product3/2
  Product/1 -> Sum/1
  Product3/1 -> Sum1/2
  Product2/1 -> Sum1/1

== system GFM_parallel_alt/SYS INV 1/VSG  Contro 1 ==
  note: Q droop Outer Control
  note: P Droop Outer Control
  Pref : Inport
  Qref : Inport  Port=2
  Pan : Inport  Port=3
  Qan : Inport  Port=4
  Gain : Gain  Gain=1/(2*H)
  Gain1 : Gain  Gain=kiq
  Gain13 : Gain  Gain=1/md
  Gain14 : Gain  Gain=nd
  Gain4 : Gain  Gain=2*pi*50
  Integrator : Integrator  InitialCondition=angle(vref_)  ContinuousStateAttributes='theta0'
  Integrator1 : Integrator
  Integrator2 : Integrator
  Step : Step  Before=1  SampleTime=0
  Step1 : Step  Time=2  Before=1  SampleTime=0
  Step2 : Step  Before=abs(vref_)  After=abs(vref_)  SampleTime=0
  Step3 : Step  Time=2  Before=1  SampleTime=0
  Step4 : Step  Time=2  After=-0.01  SampleTime=0
  Step5 : Step  Time=2.01  After=0.01  SampleTime=0
  Sum : Sum  Inputs=|+++
  Sum12 : Sum  Inputs=++|
  Sum13 : Sum  Inputs=|+-
  Sum16 : Sum  Inputs=-+-
  Sum2 : Sum  Inputs=+-
  Sum3 : Sum  Inputs=+++
  vref : Outport
  _dwt_ : Outport  Port=2
  tag scope: freqz_vsg=global
  wires:
  Qref/1 -> Sum13/1
  Sum3/1 -> vref/1
  Qan/1 -> Sum13/2
  Sum13/1 -> Gain1/1, Gain14/1
  Sum2/1 -> Gain4/1
  Gain4/1 -> Integrator/1
  Step/1 -> Sum2/2
  Step2/1 -> Sum3/1
  Sum12/1 -> [freqz_vsg], Sum2/1
  Integrator/1 -> _dwt_/1
  Gain14/1 -> Sum3/2
  Gain/1 -> Integrator1/1
  Integrator1/1 -> Gain13/1, Sum12/2
  Pref/1 -> Sum16/2
  Pan/1 -> Sum16/3
  Gain13/1 -> Sum16/1
  Step4/1 -> Sum/2
  Step3/1 -> Sum/1
  Step5/1 -> Sum/3
  Step1/1 -> Sum12/1
  Sum16/1 -> Gain/1
  Gain1/1 -> Integrator2/1
  Integrator2/1 -> Sum3/3

== system GFM_parallel_alt/SYS INV 1/VSG  Control 1 ==
  note: Q droop Outer Control
  note: P Droop Outer Control
  Pref : Inport
  Qref : Inport  Port=2
  Pan : Inport  Port=3
  Qan : Inport  Port=4
  Vpcc_lcl : Inport  Port=5
  Abs : Abs  SaturateOnIntegerOverflow=off
  Gain : Gain  Gain=1/(2*H)
  Gain1 : Gain  Gain=kiq
  Gain13 : Gain  Gain=Kd
  Gain14 : Gain  Gain=nd
  Gain4 : Gain  Gain=2*pi*50
  Integrator : Integrator  InitialCondition=angle(vref_)  ContinuousStateAttributes='theta0'
  Integrator1 : Integrator
  Integrator2 : Integrator  ContinuousStateAttributes='qdif'
  Step : Step  Before=1  SampleTime=0
  Step1 : Step  Time=2  Before=1  SampleTime=0
  Sum1 : Sum  Inputs=++|
  Sum12 : Sum  Inputs=++|
  Sum13 : Sum  Inputs=|+-
  Sum16 : Sum  Inputs=-+-
  Sum2 : Sum  Inputs=+-
  Sum3 : Sum  Inputs=++|
  vref : Outport
  _dwt_ : Outport  Port=2
  tag scope: freqz1=global
  wires:
  Qref/1 -> Sum13/1
  Sum3/1 -> vref/1
  Qan/1 -> Sum13/2
  Sum13/1 -> Gain1/1, Gain14/1
  Sum2/1 -> Gain4/1
  Gain4/1 -> Integrator/1
  Step/1 -> Sum2/2
  Sum12/1 -> [freqz1], Sum2/1
  Integrator/1 -> _dwt_/1
  Sum16/1 -> Gain/1
  Gain/1 -> Integrator1/1
  Integrator1/1 -> Gain13/1, Sum12/2
  Pref/1 -> Sum16/2
  Pan/1 -> Sum16/3
  Gain13/1 -> Sum16/1
  Step1/1 -> Sum12/1
  Gain14/1 -> Sum1/2
  Sum1/1 -> Sum3/2
  Gain1/1 -> Integrator2/1
  Integrator2/1 -> Sum1/1
  Vpcc_lcl/1 -> Abs/1
  Abs/1 -> [vpcc_abs]
  [vpcc_abs] -> Sum3/1

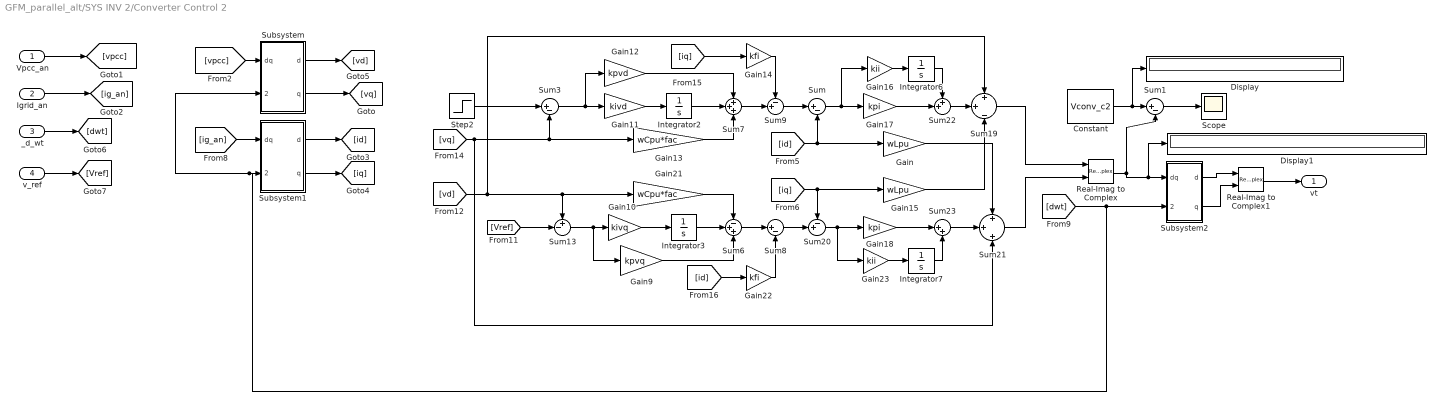
== system GFM_parallel_alt/SYS INV 2/Converter Control 2 ==
  Vpcc_an : Inport
  Igrid_an : Inport  Port=2
  _d_wt : Inport  Port=3
  v_ref : Inport  Port=4
  Constant : Constant  Value=Vconv_c2
  Display : Display
  Display1 : Display
  Gain : Gain  Gain=wLpu
  Gain10 : Gain  Gain=kivq
  Gain11 : Gain  Gain=kivd
  Gain12 : Gain  Gain=kpvd
  Gain13 : Gain  Gain=wCpu*fac
  Gain14 : Gain  Gain=kfi
  Gain15 : Gain  Gain=wLpu
  Gain16 : Gain  Gain=kii
  Gain17 : Gain  Gain=kpi
  Gain18 : Gain  Gain=kpi
  Gain21 : Gain  Gain=wCpu*fac
  Gain22 : Gain  Gain=kfi
  Gain23 : Gain  Gain=kii
  Gain9 : Gain  Gain=kpvq
  Integrator2 : Integrator  InitialCondition=PsiP2  ContinuousStateAttributes='psi_alpha2'
  Integrator3 : Integrator  InitialCondition=PsiV2  ContinuousStateAttributes='psiV2'
  Integrator6 : Integrator  InitialCondition=PsiId2  ContinuousStateAttributes='psi_id2'
  Integrator7 : Integrator  InitialCondition=PsiIq2  ContinuousStateAttributes='psi_iq2'
  Real-Imag to Complex : RealImagToComplex
  Real-Imag to Complex1 : RealImagToComplex
  Scope : Scope
  Step2 : Step  After=0  SampleTime=0
  Subsystem : Subsystem
  Subsystem1 : Subsystem
  Subsystem2 : Subsystem
  Sum{,1,3,8} (4 alike) : Sum  Inputs=|+-
  Sum13 : Sum  Inputs=+-|
  Sum19 : Sum  Inputs=+|+|-
  Sum20 : Sum  Inputs=-+|
  Sum21 : Sum  Inputs=+|+|+
  Sum22 : Sum  Inputs=++|
  Sum23 : Sum  Inputs=|++
  Sum6 : Sum  Inputs=-++
  Sum7 : Sum  Inputs=+++
  Sum9 : Sum  Inputs=-+|
  vt : Outport
  wires:
  Integrator3/1 -> Sum6/2
  Gain11/1 -> Integrator2/1
  Subsystem/2(q) -> [vq]
  Sum13/1 -> Gain10/1, Gain9/1
  Igrid_an/1 -> [ig_an]
  [vpcc] -> Subsystem/1(dq)
  Subsystem2/2(q) -> Real-Imag to Complex1/2
  Subsystem2/1(d) -> Real-Imag to Complex1/1
  [id] -> Sum/2, Gain/1
  Subsystem1/1(d) -> [id]
  [iq] -> Gain15/1, Sum20/1
  Sum21/1 -> Real-Imag to Complex/2
  Integrator6/1 -> Sum22/1
  Sum20/1 -> Gain23/1, Gain18/1
  Gain23/1 -> Integrator7/1
  Gain18/1 -> Sum23/1
  Sum22/1 -> Sum19/2
  Gain22/1 -> Sum8/2
  Gain10/1 -> Integrator3/1
  Gain14/1 -> Sum9/1
  Sum7/1 -> Sum9/2
  [ig_an] -> Subsystem1/1(dq)
  Gain13/1 -> Sum7/3
  Sum19/1 -> Real-Imag to Complex/1
  Sum3/1 -> Gain12/1, Gain11/1
  Gain16/1 -> Integrator6/1
  Sum/1 -> Gain16/1, Gain17/1
  Gain/1 -> Sum21/1
  [Vref] -> Sum13/2
  Gain9/1 -> Sum6/3
  Gain21/1 -> Sum6/1
  Subsystem1/2(q) -> [iq]
  Integrator7/1 -> Sum23/2
  Sum23/1 -> Sum21/2
  Subsystem/1(d) -> [vd]
  [vq] -> Sum3/2, Gain13/1, Sum21/3
  Gain15/1 -> Sum19/3
  [vd] -> Gain21/1, Sum13/1, Sum19/1
  Gain17/1 -> Sum22/2
  [id] -> Gain22/1
  [iq] -> Gain14/1
  Vpcc_an/1 -> [vpcc]
  Gain12/1 -> Sum7/1
  Sum6/1 -> Sum8/1
  Integrator2/1 -> Sum7/2
  Real-Imag to Complex1/1 -> vt/1
  [dwt] -> Subsystem1/2(delta_wt), Subsystem/2(delta_wt), Subsystem2/2(d_wt)
  Step2/1 -> Sum3/1
  _d_wt/1 -> [dwt]
  v_ref/1 -> [Vref]
  Real-Imag to Complex/1 -> Display1/1, Subsystem2/1(dq), Sum1/2
  Constant/1 -> Display/1, Sum1/1
  Sum1/1 -> Scope/1
  Sum9/1 -> Sum/1
  Sum8/1 -> Sum20/2

== system GFM_parallel_alt/SYS INV 2/Droop  Control 2 ==
  note: Q droop Outer Control
  note: P Droop Outer Control
  Pref : Inport
  Qref : Inport  Port=2
  Pan : Inport  Port=3
  Qan : Inport  Port=4
  Vpcc_lcl : Inport  Port=5
  Abs : Abs  SaturateOnIntegerOverflow=off
  Gain : Gain  Gain=kiq
  Gain13 : Gain  Gain=md
  Gain14 : Gain  Gain=nd
  Gain4 : Gain  Gain=2*pi*50
  Integrator : Integrator  InitialCondition=angle(vref_)  ContinuousStateAttributes='theta0_dr_2'
  Integrator1 : Integrator
  Step : Step  Before=1.00  After=1.000  SampleTime=0
  Step1 : Step  Before=abs(vref_)  After=abs(vref_)  SampleTime=0
  Step5 : Step  Time=2  Before=1  SampleTime=0
  Sum1 : Sum  Inputs=++|
  Sum12 : Sum  Inputs=++|
  Sum13 : Sum  Inputs=|+-
  Sum16 : Sum  Inputs=|+-
  Sum2 : Sum  Inputs=+-
  Sum3 : Sum  Inputs=++|
  vref : Outport
  _dwt_ : Outport  Port=2
  tag scope: freqz2=global
  wires:
  Gain13/1 -> Sum12/2
  Qref/1 -> Sum13/1
  Sum3/1 -> vref/1
  Qan/1 -> Sum13/2
  Pref/1 -> Sum16/1
  Pan/1 -> Sum16/2
  Sum13/1 -> Gain/1, Gain14/1
  Sum2/1 -> Gain4/1
  Gain4/1 -> Integrator/1
  Sum12/1 -> Sum2/1, [freqz2]
  Integrator/1 -> _dwt_/1
  Sum16/1 -> Gain13/1
  Step5/1 -> Sum12/1
  Step/1 -> Sum2/2
  Gain/1 -> Integrator1/1
  Gain14/1 -> Sum1/2
  Integrator1/1 -> Sum1/1
  Sum1/1 -> Sum3/2
  Vpcc_lcl/1 -> Abs/1
  Abs/1 -> [vpcc_abs]
  [vpcc_abs] -> Sum3/1

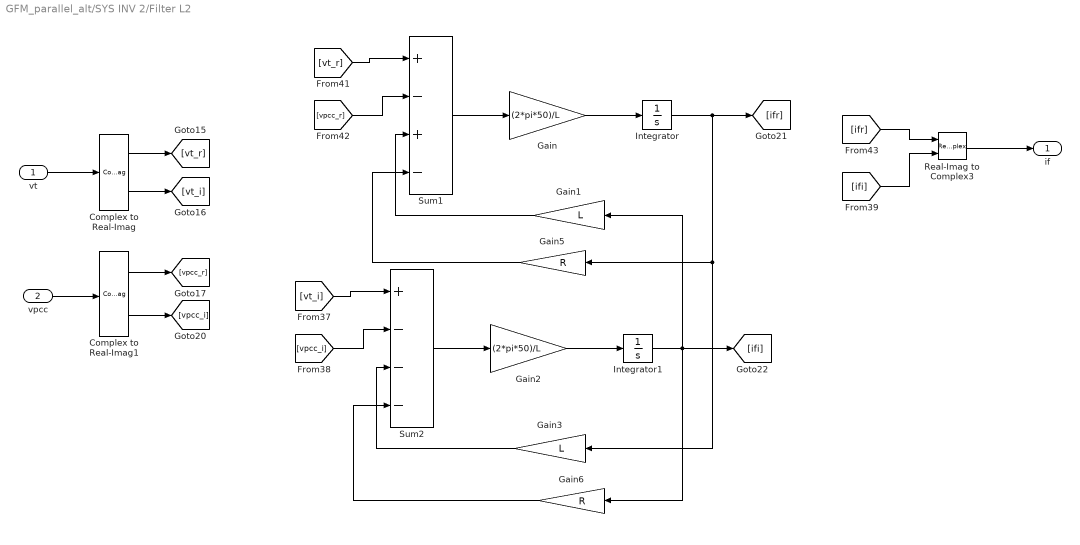
== system GFM_parallel_alt/SYS INV 2/Filter L2 ==
  "vt " : Inport
  "vpcc " : Inport  Port=2
  Complex to Real-Imag : ComplexToRealImag
  Complex to Real-Imag1 : ComplexToRealImag
  Gain : Gain  Gain=(2*pi*50)/L
  Gain1 : Gain  Gain=L
  Gain2 : Gain  Gain=(2*pi*50)/L
  Gain3 : Gain  Gain=L
  Gain5 : Gain  Gain=R
  Gain6 : Gain  Gain=R
  Integrator : Integrator  InitialCondition=real(i0)  ContinuousStateAttributes='ig2_re'
  Integrator1 : Integrator  InitialCondition=imag(i0)  ContinuousStateAttributes='ig2_im'
  Real-Imag to Complex3 : RealImagToComplex
  Sum1 : Sum  Inputs=+-+-
  Sum2 : Sum  Inputs=+---
  if : Outport
  wires:
  "vpcc "/1 -> Complex to Real-Imag1/1
  Gain5/1 -> Sum1/4
  Real-Imag to Complex3/1 -> if/1
  Integrator1/1 -> Gain6/1, Gain1/1, [ifi]
  [ifr] -> Real-Imag to Complex3/1
  "vt "/1 -> Complex to Real-Imag/1
  Integrator/1 -> Gain5/1, Gain3/1, [ifr]
  [ifi] -> Real-Imag to Complex3/2
  [vpcc_r] -> Sum1/2
  Gain6/1 -> Sum2/4
  Complex to Real-Imag/1 -> [vt_r]
  Gain1/1 -> Sum1/3
  Complex to Real-Imag/2 -> [vt_i]
  Complex to Real-Imag1/1 -> [vpcc_r]
  Sum2/1 -> Gain2/1
  Gain2/1 -> Integrator1/1
  [vt_i] -> Sum2/1
  [vpcc_i] -> Sum2/2
  [vt_r] -> Sum1/1
  Gain3/1 -> Sum2/3
  Complex to Real-Imag1/2 -> [vpcc_i]
  Gain/1 -> Integrator/1
  Sum1/1 -> Gain/1

== system GFM_parallel_alt/SYS INV 2/Filter RcLc ==
  "Vt " : Inport
  "Vlcl " : Inport  Port=2
  Complex to Real-Imag : ComplexToRealImag
  Complex to Real-Imag1 : ComplexToRealImag
  Gain : Gain  Gain=(2*pi*50)/L
  Gain1 : Gain  Gain=L
  Gain2 : Gain  Gain=(2*pi*50)/L
  Gain3 : Gain  Gain=L
  Gain5 : Gain  Gain=R
  Gain6 : Gain  Gain=R
  Integrator : Integrator  InitialCondition=real(i0)  ContinuousStateAttributes='ic2_re'
  Integrator1 : Integrator  InitialCondition=imag(i0)  ContinuousStateAttributes='ic2_im'
  Real-Imag to Complex3 : RealImagToComplex
  Sum1 : Sum  Inputs=+-+-
  Sum2 : Sum  Inputs=+---
  if : Outport
  wires:
  "Vlcl "/1 -> Complex to Real-Imag1/1
  Gain5/1 -> Sum1/4
  Real-Imag to Complex3/1 -> if/1
  Integrator1/1 -> Gain6/1, Gain1/1, [ifi]
  [ifr] -> Real-Imag to Complex3/1
  "Vt "/1 -> Complex to Real-Imag/1
  Integrator/1 -> Gain5/1, Gain3/1, [ifr]
  [ifi] -> Real-Imag to Complex3/2
  [vpcc_r] -> Sum1/2
  Gain6/1 -> Sum2/4
  Complex to Real-Imag/1 -> [vt_r]
  Gain1/1 -> Sum1/3
  Complex to Real-Imag/2 -> [vt_i]
  Complex to Real-Imag1/1 -> [vpcc_r]
  Sum2/1 -> Gain2/1
  Gain2/1 -> Integrator1/1
  [vt_i] -> Sum2/1
  [vpcc_i] -> Sum2/2
  [vt_r] -> Sum1/1
  Gain3/1 -> Sum2/3
  Complex to Real-Imag1/2 -> [vpcc_i]
  Gain/1 -> Integrator/1
  Sum1/1 -> Gain/1

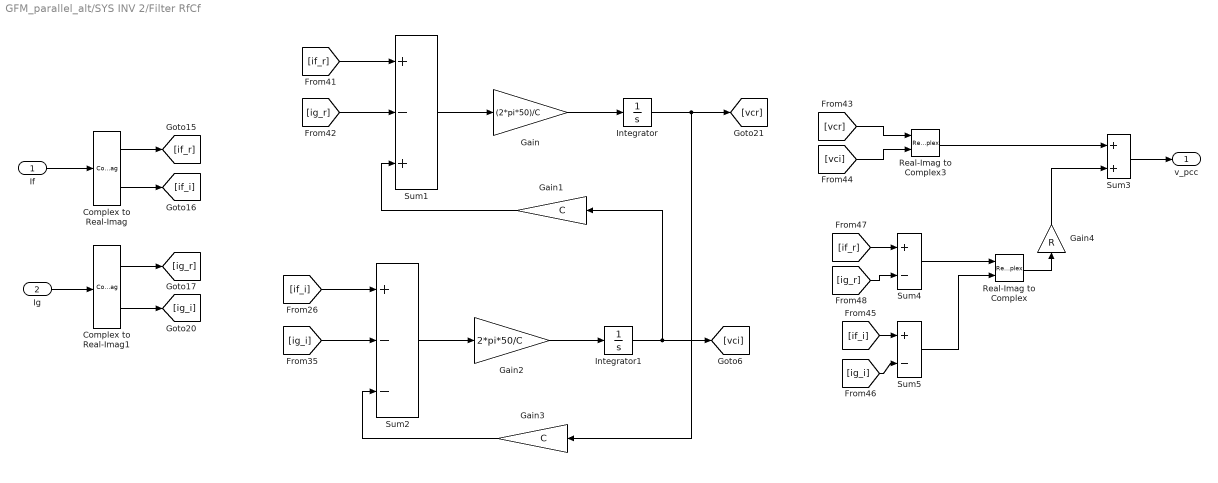
== system GFM_parallel_alt/SYS INV 2/Filter RfCf ==
  "If " : Inport
  "Ig " : Inport  Port=2
  Complex to Real-Imag : ComplexToRealImag
  Complex to Real-Imag1 : ComplexToRealImag
  Gain : Gain  Gain=(2*pi*50)/C
  Gain1 : Gain  Gain=C
  Gain2 : Gain  Gain=2*pi*50/C
  Gain3 : Gain  Gain=C
  Gain4 : Gain  Gain=R
  Integrator : Integrator  InitialCondition=real(vc0)  ContinuousStateAttributes='vc2_re'
  Integrator1 : Integrator  InitialCondition=imag(vc0)  ContinuousStateAttributes='vc2_im'
  Real-Imag to Complex : RealImagToComplex
  Real-Imag to Complex3 : RealImagToComplex
  Sum1 : Sum  Inputs=+-+
  Sum2 : Sum  Inputs=+--
  Sum3 : Sum
  Sum4 : Sum  Inputs=+-
  Sum5 : Sum  Inputs=+-
  v_pcc : Outport
  wires:
  Sum4/1 -> Real-Imag to Complex/1
  "Ig "/1 -> Complex to Real-Imag1/1
  Complex to Real-Imag1/2 -> [ig_i]
  Integrator1/1 -> Gain1/1, [vci]
  Sum1/1 -> Gain/1
  Gain/1 -> Integrator/1
  [ig_r] -> Sum1/2
  Real-Imag to Complex/1 -> Gain4/1
  Gain3/1 -> Sum2/3
  [ig_r] -> Sum4/2
  [ig_i] -> Sum5/2
  Integrator/1 -> Gain3/1, [vcr]
  [ig_i] -> Sum2/2
  Gain2/1 -> Integrator1/1
  "If "/1 -> Complex to Real-Imag/1
  [if_i] -> Sum2/1
  [if_r] -> Sum4/1
  Sum2/1 -> Gain2/1
  [if_r] -> Sum1/1
  Gain1/1 -> Sum1/3
  Sum5/1 -> Real-Imag to Complex/2
  Sum3/1 -> v_pcc/1
  [if_i] -> Sum5/1
  Gain4/1 -> Sum3/2
  Complex to Real-Imag/2 -> [if_i]
  [vci] -> Real-Imag to Complex3/2
  Real-Imag to Complex3/1 -> Sum3/1
  Complex to Real-Imag1/1 -> [ig_r]
  Complex to Real-Imag/1 -> [if_r]
  [vcr] -> Real-Imag to Complex3/1

== system GFM_parallel_alt/SYS INV 2/Subsystem4 ==
  V : Inport
  I : Inport  Port=2
  Complex to Real-Imag : ComplexToRealImag
  Complex to Real-Imag1 : ComplexToRealImag
  Product{,1..3} (4 alike) : Product
  Sum : Sum
  Sum1 : Sum  Inputs=-+
  P : Outport
  Q : Outport  Port=2
  wires:
  Complex to Real-Imag/1 -> Product2/1, Product/1
  Sum1/1 -> Q/1
  V/1 -> Complex to Real-Imag/1
  Complex to Real-Imag1/2 -> Product2/2, Product1/2
  Product1/1 -> Sum/2
  Sum/1 -> P/1
  I/1 -> Complex to Real-Imag1/1
  Complex to Real-Imag/2 -> Product3/1, Product1/1
  Complex to Real-Imag1/1 -> Product/2, Product3/2
  Product/1 -> Sum/1
  Product3/1 -> Sum1/2
  Product2/1 -> Sum1/1

== system GFM_parallel_alt/SYS INV 2/VSG  Control 2 ==
  note: Q droop Outer Control
  note: P Droop Outer Control
  Pref : Inport
  Qref : Inport  Port=2
  Pan : Inport  Port=3
  Qan : Inport  Port=4
  Vpcc_lcl : Inport  Port=5
  Abs : Abs  SaturateOnIntegerOverflow=off
  Gain : Gain  Gain=1/(2*H)
  Gain1 : Gain  Gain=kiq
  Gain13 : Gain  Gain=1/md
  Gain14 : Gain  Gain=nd
  Gain4 : Gain  Gain=2*pi*50
  Integrator : Integrator  InitialCondition=angle(vref_)  ContinuousStateAttributes='theta0'
  Integrator1 : Integrator  ContinuousStateAttributes='swing'
  Integrator2 : Integrator  ContinuousStateAttributes='qdif'
  Step : Step  Before=1  SampleTime=0
  Step1 : Step  Time=2  Before=1  SampleTime=0
  Sum1 : Sum  Inputs=++|
  Sum12 : Sum  Inputs=++|
  Sum13 : Sum  Inputs=|+-
  Sum16 : Sum  Inputs=-+-
  Sum2 : Sum  Inputs=+-
  Sum3 : Sum  Inputs=++|
  vref : Outport
  _dwt_ : Outport  Port=2
  tag scope: freqz2=global
  wires:
  Qref/1 -> Sum13/1
  Sum3/1 -> vref/1
  Qan/1 -> Sum13/2
  Sum13/1 -> Gain1/1, Gain14/1
  Sum2/1 -> Gain4/1
  Gain4/1 -> Integrator/1
  Step/1 -> Sum2/2
  Sum12/1 -> [freqz2], Sum2/1
  Integrator/1 -> _dwt_/1
  Sum16/1 -> Gain/1
  Gain/1 -> Integrator1/1
  Integrator1/1 -> Gain13/1, Sum12/2
  Pref/1 -> Sum16/2
  Pan/1 -> Sum16/3
  Gain13/1 -> Sum16/1
  Step1/1 -> Sum12/1
  Gain14/1 -> Sum1/2
  Sum1/1 -> Sum3/2
  Gain1/1 -> Integrator2/1
  Integrator2/1 -> Sum1/1
  Vpcc_lcl/1 -> Abs/1
  Abs/1 -> [vpcc_abs]
  [vpcc_abs] -> Sum3/1

== system GFM_parallel_alt/SYS INV 1/Converter Control 1/Subsystem ==
  dq : Inport
  delta_wt : Inport  Port=2
  Complex to Real-Imag1 : ComplexToRealImag
  Divide1 : Product  Inputs=**
  Gain6 : Gain  Gain=-1i
  Math Function : Math  SignedPower=on  RndMeth=Zero
  d : Outport
  q : Outport  Port=2
  wires:
  Math Function/1 -> Divide1/2
  Complex to Real-Imag1/1 -> d/1
  Divide1/1 -> Complex to Real-Imag1/1
  delta_wt/1 -> Gain6/1
  Gain6/1 -> Math Function/1
  dq/1 -> Divide1/1
  Complex to Real-Imag1/2 -> q/1

== system GFM_parallel_alt/SYS INV 1/Converter Control 1/Subsystem1 ==
  dq : Inport
  delta_wt : Inport  Port=2
  Complex to Real-Imag1 : ComplexToRealImag
  Divide1 : Product  Inputs=**
  Gain6 : Gain  Gain=-1i
  Math Function : Math  SignedPower=on  RndMeth=Zero
  d : Outport
  q : Outport  Port=2
  wires:
  Math Function/1 -> Divide1/2
  Complex to Real-Imag1/1 -> d/1
  Divide1/1 -> Complex to Real-Imag1/1
  delta_wt/1 -> Gain6/1
  Gain6/1 -> Math Function/1
  dq/1 -> Divide1/1
  Complex to Real-Imag1/2 -> q/1

== system GFM_parallel_alt/SYS INV 1/Converter Control 1/Subsystem2 ==
  dq : Inport
  d_wt : Inport  Port=2
  Complex to Real-Imag1 : ComplexToRealImag
  Divide1 : Product  Inputs=**
  Gain6 : Gain  Gain=1i
  Math Function : Math  SignedPower=on  RndMeth=Zero
  d : Outport
  q : Outport  Port=2
  wires:
  Complex to Real-Imag1/1 -> d/1
  Divide1/1 -> Complex to Real-Imag1/1
  d_wt/1 -> Gain6/1
  Gain6/1 -> Math Function/1
  dq/1 -> Divide1/1
  Complex to Real-Imag1/2 -> q/1
  Math Function/1 -> Divide1/2

== system GFM_parallel_alt/SYS INV 2/Converter Control 2/Subsystem ==
  dq : Inport
  delta_wt : Inport  Port=2
  Complex to Real-Imag1 : ComplexToRealImag
  Divide1 : Product  Inputs=**
  Gain6 : Gain  Gain=-1i
  Math Function : Math  SignedPower=on  RndMeth=Zero
  d : Outport
  q : Outport  Port=2
  wires:
  Math Function/1 -> Divide1/2
  Complex to Real-Imag1/1 -> d/1
  Divide1/1 -> Complex to Real-Imag1/1
  delta_wt/1 -> Gain6/1
  Gain6/1 -> Math Function/1
  dq/1 -> Divide1/1
  Complex to Real-Imag1/2 -> q/1

== system GFM_parallel_alt/SYS INV 2/Converter Control 2/Subsystem1 ==
  dq : Inport
  delta_wt : Inport  Port=2
  Complex to Real-Imag1 : ComplexToRealImag
  Divide1 : Product  Inputs=**
  Gain6 : Gain  Gain=-1i
  Math Function : Math  SignedPower=on  RndMeth=Zero
  d : Outport
  q : Outport  Port=2
  wires:
  Math Function/1 -> Divide1/2
  Complex to Real-Imag1/1 -> d/1
  Divide1/1 -> Complex to Real-Imag1/1
  delta_wt/1 -> Gain6/1
  Gain6/1 -> Math Function/1
  dq/1 -> Divide1/1
  Complex to Real-Imag1/2 -> q/1

== system GFM_parallel_alt/SYS INV 2/Converter Control 2/Subsystem2 ==
  dq : Inport
  d_wt : Inport  Port=2
  Complex to Real-Imag1 : ComplexToRealImag
  Divide1 : Product  Inputs=**
  Gain6 : Gain  Gain=1i
  Math Function : Math  SignedPower=on  RndMeth=Zero
  d : Outport
  q : Outport  Port=2
  wires:
  Complex to Real-Imag1/1 -> d/1
  Divide1/1 -> Complex to Real-Imag1/1
  d_wt/1 -> Gain6/1
  Gain6/1 -> Math Function/1
  dq/1 -> Divide1/1
  Complex to Real-Imag1/2 -> q/1
  Math Function/1 -> Divide1/2
